simulink model "Ativa_reativa_2W_R150"  (Simulink 10.1)
settings: Solver=ode23t  StartTime=0.0  StopTime=0.1  RelTol=1e-5  EnableMultiTasking=on
libraries: powerlib x9, powerlib_extras x2
settings Model: Creator=alunos  LastModifiedBy=victo
settings DataIOCC: LimitDataPoints=on  SignalLoggingSaveFormat=ModelDataLogs
settings OptimizationCC: ExpressionDepthLimit=2147483647
settings DebuggingCC: SolverPrmCheckMsg=warning  FcnCallInpInsideContextMsg=warning  StateNameClashWarn=warning

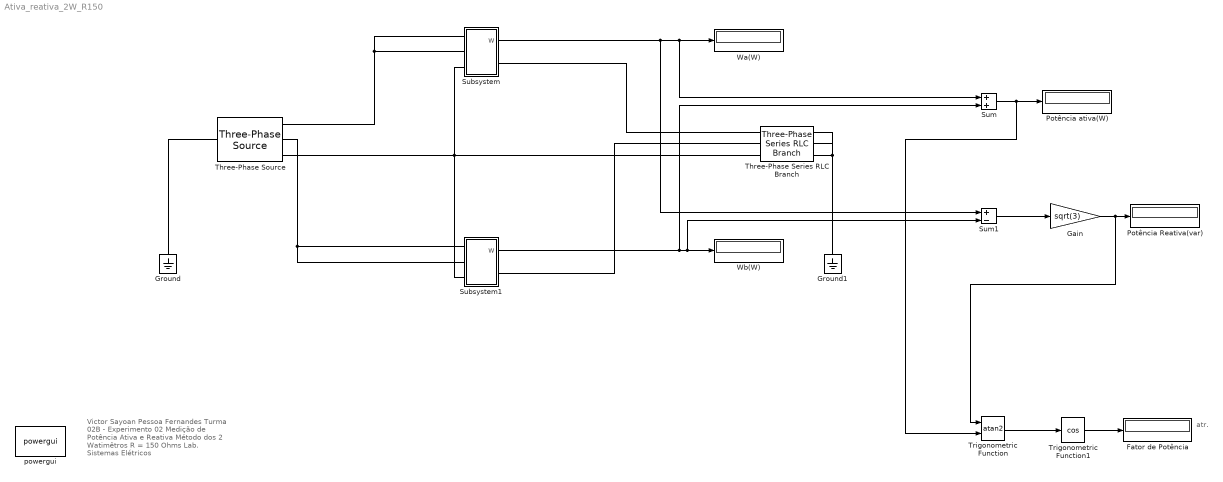
== system Ativa_reativa_2W_R150 ==
  note: atr.
  note: Victor Sayoan Pessoa Fernandes
      | Turma 02B - Experimento 02
      | Medição de Potência Ativa e Reativa
      | Método dos 2 Watimêtros
      | R = 150 Ohms
      | Lab. Sistemas Elétricos
  Fator de Potência : Display
      settings: Format=bank
  Gain : Gain  Gain=sqrt(3)
  Ground : powerlib/Elements/Ground  LConnTagsString=a
  Ground1 : powerlib/Elements/Ground  LConnTagsString=a
  Potência Reativa(var) : Display
      settings: Format=bank
  Potência ativa(W) : Display
      settings: Format=bank
  Subsystem : Subsystem
  Subsystem1 : Subsystem
  Sum : Sum
  Sum1 : Sum  Inputs=+-
  Three-Phase Series RLC Branch : powerlib/Elements/Three-Phase Series RLC Branch  LConnTagsString=A|B|C  RConnTagsString=A|B|C  BranchType=RL  Resistance=150  Inductance=300e-3  Capacitance=1e-6  Measurements=None
  Three-Phase Source : powerlib/Electrical Sources/Three-Phase Source  InternalConnection=Yn  VoltagePhases=off  Voltage=220  PhaseAngle=90  Voltage_phases=[25e3 25e3 25e3]/sqrt(3)  PhaseAngles_phases=[0 -120 +120]  Frequency=60  NonIdealSource=on  SpecifyImpedance=off  Resistance=0.001  Inductance=0  ShortCircuitLevel=100e6  BaseVoltage=25e3  XRratio=7  BusType=swing  Pref=0  Qref=0  Prefabc=[10e3, 10e3, 10e3]  Qrefabc=[0, 0, 0]  Qmin=-inf  Qmax=inf
  Trigonometric Function : Trigonometry  Operator=atan2
  Trigonometric Function1 : Trigonometry  Operator=cos
  Wa(W) : Display
      settings: Format=bank
  Wb(W) : Display
      settings: Format=bank
  powergui : powerlib/powergui  Priority=1  SimulationMode=Continuous  SampleTime=50e-6  frequency=60  Iterations=50  frequencyindice=60  Pbase=100e6  ErrMax=1e-4  UnitsV=kV  UnitsW=MW  buscounter=0  FunctionMessages=off  echomessages=off  EnableUseOfTLC=off  CurrentSourceSwitches=on  DisableSnubberDevices=off  DisableRonSwitches=off  DisableVfSwitches=off  DisplayEquations=off  AutomaticDiscreteSolvers=off  SolverType=Tustin/Backward Euler (TBE)  Interpol=off  ExternalGateDelay=off  methode=off  Ts=100  x0status=blocks  SPID=off  SwTol=0  HookPort=off  NonlinearTolerance=1e-4  nMaxIteration=100  ContinueOnMaxIteration=off  RestoreLinks=warning  ResistiveCurrentMeasurement=off  Frange=[0:2:500]  Ylog=off  Xlog=on  ShowGrid=off  save=off  variable=ZData  structure=0  ZoomFFT=off  StartTime=0.0  cycles=1  DisplayStyle=1  fundamental=60  FreqAxis=off  MaxFrequency=1000  frequencyindicesteady=1  RmsSteady=1  display=off
  wires:
  Subsystem/1(W) -> Wa(W)/1, Sum/1, Sum1/1
  Subsystem1/1(W) -> Sum/2, Wb(W)/1, Sum1/2
  Sum/1 -> Potência ativa(W)/1, Trigonometric Function/2
  Gain/1 -> Potência Reativa(var)/1, Trigonometric Function/1
  Sum1/1 -> Gain/1
  Trigonometric Function/1 -> Trigonometric Function1/1
  Trigonometric Function1/1 -> Fator de Potência/1
  connections:
  Ground/LConn1 -- Three-Phase Source/LConn1
  Three-Phase Series RLC Branch/RConn1 -- Three-Phase Series RLC Branch/RConn2 -- Three-Phase Series RLC Branch/RConn3 -- Ground1/LConn1
  Three-Phase Source/RConn3 -- Three-Phase Series RLC Branch/LConn3 -- Subsystem/LConn3 -- Subsystem1/LConn3
  Subsystem/RConn1 -- Three-Phase Series RLC Branch/LConn1
  Subsystem/LConn1 -- Three-Phase Source/RConn1 -- Subsystem/LConn2
  Subsystem1/LConn1 -- Three-Phase Source/RConn2 -- Subsystem1/LConn2
  Subsystem1/RConn1 -- Three-Phase Series RLC Branch/LConn2

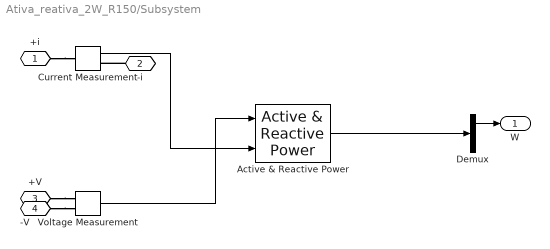
== system Ativa_reativa_2W_R150/Subsystem ==
  Active & Reactive Power : powerlib_extras/Measurements/Active & Reactive Power  f1=60
      settings: SourceProductBaseCode=PS
  Current Measurement : powerlib/Measurements/Current Measurement  PhasorSimulation=off  OutputType=Complex  PSBequivalent=0
  Demux : Demux  Outputs=2
  Voltage Measurement : powerlib/Measurements/Voltage Measurement  PhasorSimulation=off  OutputType=Complex  PSBequivalent=0
  +i : PMIOPort  Side=Left
  -i : PMIOPort  Port=2  Side=Right
  +V : PMIOPort  Port=3  Side=Left
  -V : PMIOPort  Port=4  Side=Left
  W : Outport
  wires:
  Current Measurement/1 -> Active & Reactive Power/2
  Voltage Measurement/1 -> Active & Reactive Power/1
  Active & Reactive Power/1 -> Demux/1
  Demux/1 -> W/1
  connections:
  +i/RConn1 -- Current Measurement/LConn1
  -i/RConn1 -- Current Measurement/RConn1
  +V/RConn1 -- Voltage Measurement/LConn1
  -V/RConn1 -- Voltage Measurement/LConn2

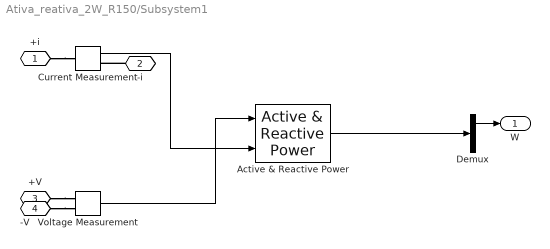
== system Ativa_reativa_2W_R150/Subsystem1 ==
  Active & Reactive Power : powerlib_extras/Measurements/Active & Reactive Power  f1=60
      settings: SourceProductBaseCode=PS
  Current Measurement : powerlib/Measurements/Current Measurement  PhasorSimulation=off  OutputType=Complex  PSBequivalent=0
  Demux : Demux  Outputs=2
  Voltage Measurement : powerlib/Measurements/Voltage Measurement  PhasorSimulation=off  OutputType=Complex  PSBequivalent=0
  +i : PMIOPort  Side=Left
  -i : PMIOPort  Port=2  Side=Right
  +V : PMIOPort  Port=3  Side=Left
  -V : PMIOPort  Port=4  Side=Left
  W : Outport
  wires:
  Current Measurement/1 -> Active & Reactive Power/2
  Voltage Measurement/1 -> Active & Reactive Power/1
  Active & Reactive Power/1 -> Demux/1
  Demux/1 -> W/1
  connections:
  +i/RConn1 -- Current Measurement/LConn1
  -i/RConn1 -- Current Measurement/RConn1
  +V/RConn1 -- Voltage Measurement/LConn1
  -V/RConn1 -- Voltage Measurement/LConn2
